simulink model "mc_att_control"  (R2024b)
settings: configuration reference "simulation" (kept outside this file)
undefined symbols (not defined in the file or in its folder): AIRMODE_ROLL_PITCH_YAW, deg, DiscIntNeverNeededParam, MC_ACRO_EXPO, MC_ACRO_EXPO_Y, MC_ACRO_P_MAX, MC_ACRO_R_MAX, MC_ACRO_SUPEXPO, MC_ACRO_SUPEXPOY, MC_ACRO_Y_MAX, MC_AIRMODE, MC_BAT_SCALE_EN, MC_MAN_TILT_TAU, MC_PITCH_P, MC_PITCHRATE_D, MC_PITCHRATE_FF, MC_PITCHRATE_I, MC_PITCHRATE_K, MC_PITCHRATE_MAX, MC_PITCHRATE_P, MC_PR_INT_LIM, MC_ROLL_P, MC_ROLLRATE_D, MC_ROLLRATE_FF, MC_ROLLRATE_I, MC_ROLLRATE_K, MC_ROLLRATE_MAX, MC_ROLLRATE_P, MC_RR_INT_LIM, MC_YAW_P, MC_YAW_WEIGHT, MC_YAWRATE_D, MC_YAWRATE_FF, MC_YAWRATE_I, MC_YAWRATE_K, MC_YAWRATE_MAX, MC_YAWRATE_P, MC_YR_INT_LIM, MPC_MAN_TILT_MAX, MPC_MAN_Y_MAX, MPC_MANTHR_MIN, MPC_THR_CURVE, MPC_THR_HOVER, MPC_THR_MAX, param_mpc_thr_hover, param_mpc_thr_max, rad, s, VEHICLE_TYPE_ROTARY_WING
libraries: simulink x22, aerolibutil x11, sharedtransform x4, aerolibconvert2 x3, vrlib x2, sharedutil x1
(part 1 of 2)
settings Model: DataDictionary=nextpilot_datadict.sldd  Creator=DELL  LastModifiedBy=93114
settings ConfigSetRef: SourceName=simulation

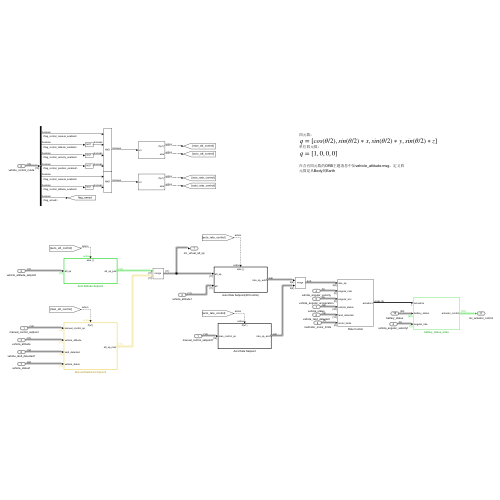
[thumbnail: Simulink's stored preview of the top-level diagram]
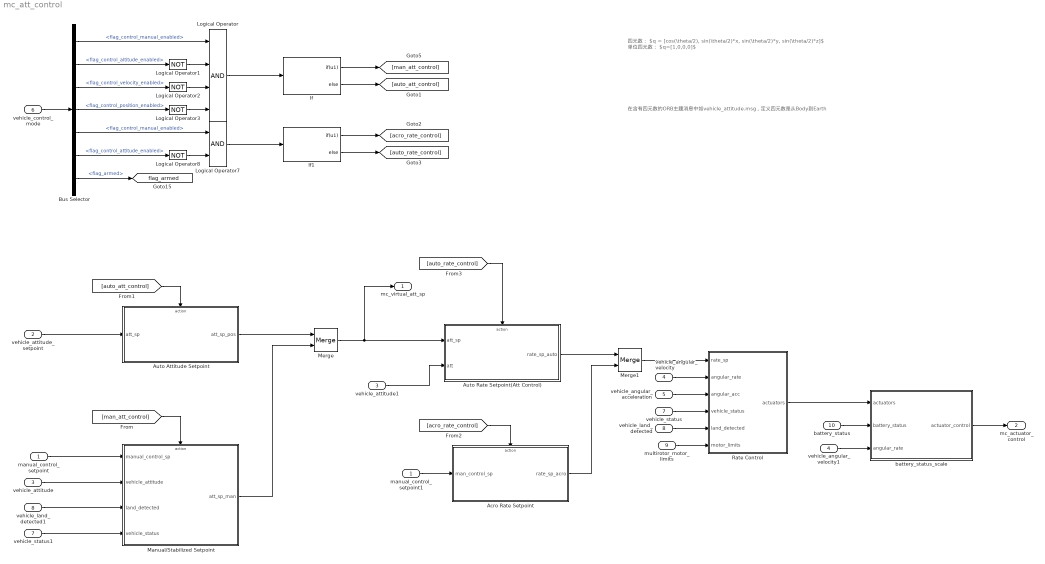
== system mc_att_control ==
  note: 在含有四元数的ORB主题消息中如vehicle_attitude.msg，定义四元数是从Body到Earth
  note: 四元数：
      | $q = [cos(\theta/2), sin(\theta/2)*x, sin(\theta/2)*y, sin(\theta/2)*z]$
      | 单位四元数：
      | $q=[1,0,0,0]$
  manual_control_setpoint : Inport  OutDataTypeStr=Bus: manual_control_setpoint_s
  vehicle_attitude_setpoint : Inport  Port=2  OutDataTypeStr=Bus: vehicle_attitude_setpoint_s
  vehicle_attitude : Inport  Port=3  OutDataTypeStr=Bus: vehicle_attitude_s
  vehicle_angular_velocity : Inport  Port=4  OutDataTypeStr=Bus: vehicle_angular_velocity_s
  vehicle_angular_acceleration : Inport  Port=5  OutDataTypeStr=Bus: vehicle_angular_acceleration_s
  vehicle_control_mode : Inport  Port=6  OutDataTypeStr=Bus: vehicle_control_mode_s
  vehicle_status : Inport  Port=7  OutDataTypeStr=Bus: vehicle_status_s
  vehicle_land_detected : Inport  Port=8  OutDataTypeStr=Bus: vehicle_land_detected_s
  multirotor_motor_limits : Inport  Port=9  OutDataTypeStr=Bus: multirotor_motor_limits_s
  battery_status : Inport  Port=10  OutDataTypeStr=Bus: battery_status_s
  Acro Rate Setpoint : Subsystem
  Auto Attitude Setpoint : Subsystem
  Auto Rate Setpoint(Att Control) : Subsystem
  Bus Selector : BusSelector  OutputSignals=flag_control_manual_enabled,flag_control_altitude_enabled,flag_control_velocity_enabled,flag_control_position_enabled,flag_control_manual_enabled,flag_control_attitude_enabled,flag_armed
  If : If  IfExpression=u1
  If1 : If  IfExpression=u1
  Logical Operator : Logic  Inputs=4  AllPortsSameDT=off  OutDataTypeStr=boolean
  Logical Operator{1..3,8} (4 alike) : Logic  Operator=NOT  Inputs=4  AllPortsSameDT=off  OutDataTypeStr=boolean
  Logical Operator7 : Logic  AllPortsSameDT=off  OutDataTypeStr=boolean
  Manual/Stabilized Setpoint : Subsystem
  Merge : Merge
  Merge1 : Merge
  Rate Control : Subsystem
  battery_status_scale : Subsystem
  manual_control_setpoint1 : InportShadow  OutDataTypeStr=Bus: manual_control_setpoint_s
  vehicle_angular_velocity1 : InportShadow  Port=4  OutDataTypeStr=Bus: vehicle_angular_velocity_s
  vehicle_attitude1 : InportShadow  Port=3  OutDataTypeStr=Bus: vehicle_attitude_s
  vehicle_land_detected1 : InportShadow  Port=8  OutDataTypeStr=Bus: vehicle_land_detected_s
  vehicle_status1 : InportShadow  Port=7  OutDataTypeStr=Bus: vehicle_status_s
  mc_virtual_att_sp : Outport  OutDataTypeStr=Bus: vehicle_attitude_setpoint_s  BusOutputAsStruct=on
  mc_actuator_control : Outport  Port=2  OutDataTypeStr=Bus: actuator_controls_s  BusOutputAsStruct=on
  tag scope: flag_armed=global
  wires:
  manual_control_setpoint/1 -> Manual/Stabilized Setpoint/1(manual_control_sp)
  Bus Selector/1 -> Logical Operator/1  "<flag_control_manual_enabled>"
  Bus Selector/2 -> Logical Operator1/1  "<flag_control_altitude_enabled>"
  Bus Selector/3 -> Logical Operator2/1  "<flag_control_velocity_enabled>"
  Bus Selector/4 -> Logical Operator3/1  "<flag_control_position_enabled>"
  Logical Operator1/1 -> Logical Operator/2
  Logical Operator2/1 -> Logical Operator/3
  Logical Operator3/1 -> Logical Operator/4
  vehicle_attitude/1 -> Manual/Stabilized Setpoint/2(vehicle_attitude)
  Logical Operator8/1 -> Logical Operator7/2
  Logical Operator7/1 -> If1/1
  Auto Rate Setpoint(Att Control)/1(rate_sp_auto) -> Merge1/1
  Manual/Stabilized Setpoint/1(att_sp_man) -> Merge/2
  vehicle_attitude1/1 -> Auto Rate Setpoint(Att Control)/2(att)
  vehicle_land_detected1/1 -> Manual/Stabilized Setpoint/3(land_detected)
  If/1 -> [man_att_control]
  If/2 -> [auto_att_control]
  [man_att_control] -> Manual/Stabilized Setpoint/Action
  [auto_att_control] -> Auto Attitude Setpoint/Action
  vehicle_control_mode/1 -> Bus Selector/1
  If1/1 -> [acro_rate_control]
  If1/2 -> [auto_rate_control]
  [acro_rate_control] -> Acro Rate Setpoint/Action
  Bus Selector/5 -> Logical Operator7/1  "<flag_control_manual_enabled>"
  Bus Selector/6 -> Logical Operator8/1  "<flag_control_attitude_enabled>"
  Bus Selector/7 -> [flag_armed]  "<flag_armed>"
  vehicle_status/1 -> Rate Control/4(vehicle_status)
  vehicle_status1/1 -> Manual/Stabilized Setpoint/4(vehicle_status)
  manual_control_setpoint1/1 -> Acro Rate Setpoint/1(man_control_sp)
  vehicle_angular_velocity/1 -> Rate Control/2(angular_rate)
  vehicle_angular_acceleration/1 -> Rate Control/3(angular_acc)
  Acro Rate Setpoint/1(rate_sp_acro) -> Merge1/2
  [auto_rate_control] -> Auto Rate Setpoint(Att Control)/Action
  Merge1/1 -> Rate Control/1(rate_sp)
  Merge/1 -> mc_virtual_att_sp/1, Auto Rate Setpoint(Att Control)/1(att_sp)
  battery_status_scale/1(actuator_control) -> mc_actuator_control/1
  Rate Control/1(actuators) -> battery_status_scale/1(actuators)
  battery_status/1 -> battery_status_scale/2(battery_status)
  vehicle_angular_velocity1/1 -> battery_status_scale/3(angular_rate)
  Auto Attitude Setpoint/1(att_sp_pos) -> Merge/1
  vehicle_attitude_setpoint/1 -> Auto Attitude Setpoint/1(att_sp)
  Logical Operator/1 -> If/1
  multirotor_motor_limits/1 -> Rate Control/6(motor_limits)
  vehicle_land_detected/1 -> Rate Control/5(land_detected)

== system mc_att_control/Acro Rate Setpoint ==
  Bus Element In : Inport  PortName=man_control_sp
  Bus Element In1 : Inport  PortName=man_control_sp  Element=z
  Action Port : ActionPort  ActionPortLabel=if(u1)
  Angular Velocity Conversion : aerolibconvert2/Angular Velocity Conversion  IU=deg/s  OU=rad/s
  Constant : Constant  Value=MC_ACRO_R_MAX
  Constant1 : Constant  Value=MC_ACRO_P_MAX
  Constant2 : Constant  Value=MC_ACRO_Y_MAX
  Demux : Demux  Outputs=3
  Gain : Gain
  Gain1 : Gain
  Gain2 : Gain
  Mux : Mux  Inputs=3
  Product : Product
  Saturation : Saturate  UpperLimit=1.0  LowerLimit=0.0
      settings: AttributesFormatString=[%<LowerLimit>,%<UpperLimit>]
  Unary Minus : UnaryMinus
  superexpo : Subsystem
  Bus Element Out : Outport  PortName=rate_sp_acro  Element=roll_rate_sp
  Bus Element Out1 : Outport  PortName=rate_sp_acro  Element=pitch_rate_sp
  Bus Element Out2 : Outport  PortName=rate_sp_acro  Element=yaw_rate_sp
  Bus Element Out3 : Outport  PortName=rate_sp_acro  Element=thrust_sp
  wires:
  Bus Element In1/1 -> Saturation/1
  Saturation/1 -> Unary Minus/1
  superexpo/1(man_rate_sp) -> Product/1
  Constant1/1 -> Mux/2
  Constant/1 -> Mux/1
  Constant2/1 -> Mux/3
  Mux/1 -> Angular Velocity Conversion/1
  Angular Velocity Conversion/1 -> Product/2  "parameter"
  Bus Element In/1 -> superexpo/1(man_stick)
  Demux/1 -> Gain2/1
  Demux/2 -> Gain1/1
  Demux/3 -> Gain/1
  Unary Minus/1 -> Bus Element Out3/1
  Product/1 -> Demux/1
  Gain/1 -> Bus Element Out2/1
  Gain1/1 -> Bus Element Out1/1
  Gain2/1 -> Bus Element Out/1

== system mc_att_control/Auto Attitude Setpoint ==
  att_sp : Inport
  Action Port : ActionPort  ActionPortLabel=else
  att_sp_pos : Outport
  wires:
  att_sp/1 -> att_sp_pos/1

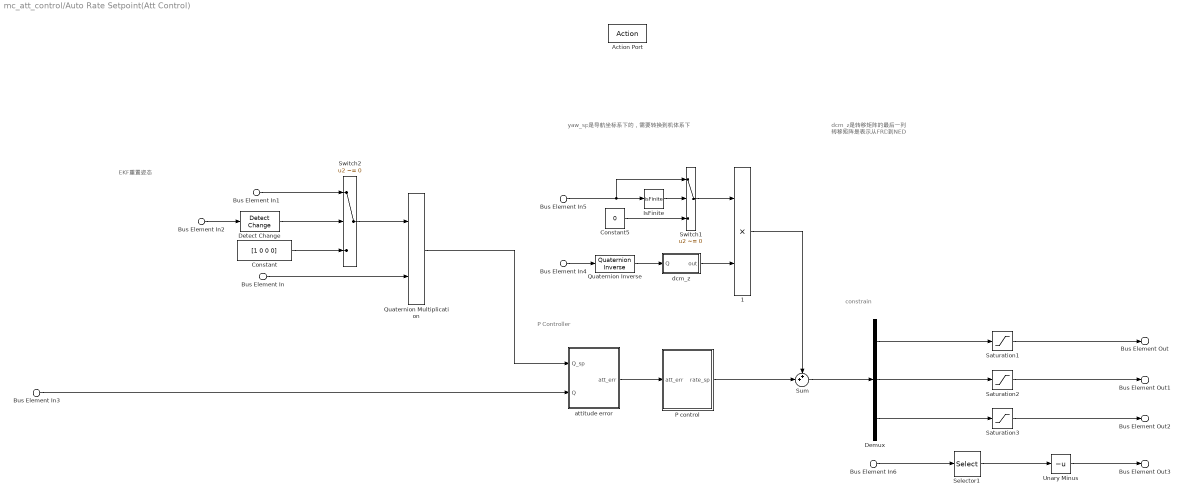
== system mc_att_control/Auto Rate Setpoint(Att Control) ==
  note: dcm_z是转移矩阵的最后一列
      | 转移矩阵是表示从FRD到NED
  note: constrain
  note: yaw_sp是导航坐标系下的，需要转换到机体系下
  note: EKF重置姿态
  note: P Controller
  Bus Element In : Inport  PortName=att_sp  Element=q_d
  Bus Element In5 : Inport  PortName=att_sp  Element=yaw_sp_move_rate
  Bus Element In6 : Inport  PortName=att_sp  Element=thrust_body
  Bus Element In1 : Inport  Port=2  PortName=att  Element=delta_q_reset
  Bus Element In2 : Inport  Port=2  PortName=att  Element=quat_reset_counter
  Bus Element In3 : Inport  Port=2  PortName=att  Element=q
  Bus Element In4 : Inport  Port=2  PortName=att  Element=q
  Action Port : ActionPort  ActionPortLabel=else
  1 : Product
  Constant : Constant  Value=[1 0 0 0]  OutDataTypeStr=single
  Constant5 : Constant  Value=0  OutDataTypeStr=single
  Demux : Demux  Outputs=3
  Detect Change : simulink/Logic and Bit Operations/Detect Change  vinit=0  OutDataTypeStr=boolean
  IsFinite : RelationalOperator  Operator=isFinite  OutDataTypeStr=boolean  RndMeth=Simplest  InputSameDT=off
  P control : Subsystem
  Quaternion Inverse : aerolibutil/Quaternion Inverse
  Quaternion Multiplication : aerolibutil/Quaternion Multiplication
  Saturation1 : Saturate  UpperLimit=deg2rad(MC_ROLLRATE_MAX)  LowerLimit=-deg2rad(MC_ROLLRATE_MAX)
      settings: AttributesFormatString=[%<LowerLimit>,%<UpperLimit>]
  Saturation2 : Saturate  UpperLimit=deg2rad(MC_PITCHRATE_MAX)  LowerLimit=-deg2rad(MC_PITCHRATE_MAX)
      settings: AttributesFormatString=[%<LowerLimit>,%<UpperLimit>]
  Saturation3 : Saturate  UpperLimit=deg2rad(MC_YAWRATE_MAX)  LowerLimit=-deg2rad(MC_YAWRATE_MAX)
      settings: AttributesFormatString=[%<LowerLimit>,%<UpperLimit>]
  Selector1 : Selector  InputPortWidth=3  IndexOptions=Index vector (dialog)  Indices=3  OutputSizes=1
  Sum : Sum  Inputs=++|
  Switch1 : Switch  Criteria=u2 ~= 0  SaturateOnIntegerOverflow=off  InputSameDT=off
  Switch2 : Switch  Criteria=u2 ~= 0  SaturateOnIntegerOverflow=off  InputSameDT=off
  Unary Minus : UnaryMinus
  attitude error : Subsystem
  dcm_z : Subsystem
  Bus Element Out : Outport  PortName=rate_sp_auto  Element=roll_rate_sp
  Bus Element Out1 : Outport  PortName=rate_sp_auto  Element=pitch_rate_sp
  Bus Element Out2 : Outport  PortName=rate_sp_auto  Element=yaw_rate_sp
  Bus Element Out3 : Outport  PortName=rate_sp_auto  Element=thrust_sp
  wires:
  P control/1(rate_sp) -> Sum/2
  Demux/1 -> Saturation1/1
  Demux/2 -> Saturation2/1
  Demux/3 -> Saturation3/1
  Saturation1/1 -> Bus Element Out/1
  Saturation2/1 -> Bus Element Out1/1
  Saturation3/1 -> Bus Element Out2/1
  Quaternion Multiplication/1 -> attitude error/1(Q_sp)
  Bus Element In3/1 -> attitude error/2(Q)
  Bus Element In4/1 -> Quaternion Inverse/1
  Quaternion Inverse/1 -> dcm_z/1(Q)
  dcm_z/1(out) -> 1/2
  Bus Element In5/1 -> Switch1/1, IsFinite/1
  1/1 -> Sum/1
  IsFinite/1 -> Switch1/2
  Constant5/1 -> Switch1/3
  Switch1/1 -> 1/1
  Detect Change/1 -> Switch2/2
  Switch2/1 -> Quaternion Multiplication/1
  Bus Element In/1 -> Quaternion Multiplication/2
  Constant/1 -> Switch2/3
  Bus Element In2/1 -> Detect Change/1
  Bus Element In1/1 -> Switch2/1
  Bus Element In6/1 -> Selector1/1
  Unary Minus/1 -> Bus Element Out3/1
  Sum/1 -> Demux/1
  Selector1/1 -> Unary Minus/1
  attitude error/1(att_err) -> P control/1(att_err)

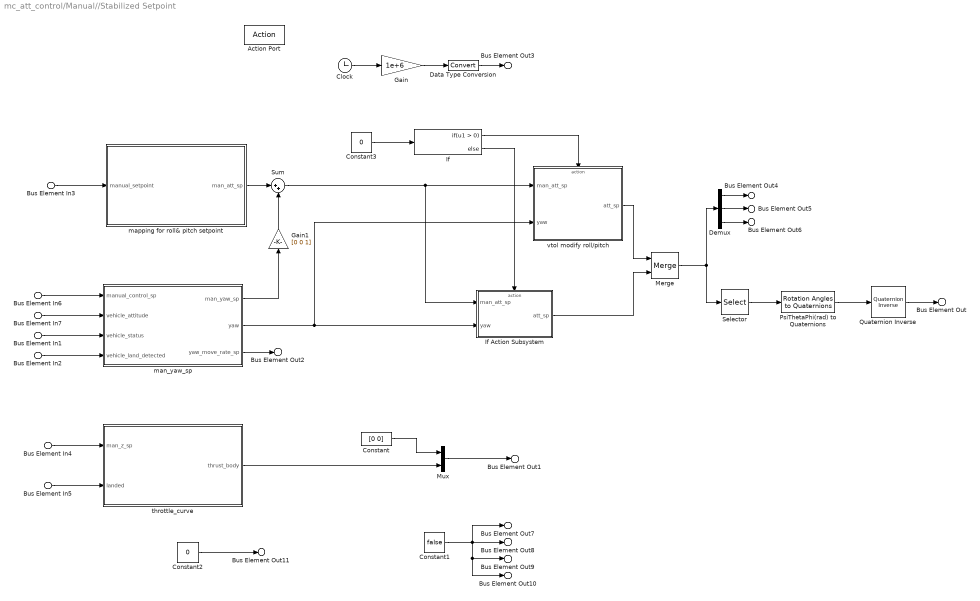
== system mc_att_control/Manual//Stabilized Setpoint ==
  Bus Element In6 : Inport  PortName=manual_control_sp
  Bus Element In3 : Inport  PortName=manual_control_sp
  Bus Element In4 : Inport  PortName=manual_control_sp  Element=z
  Bus Element In7 : Inport  Port=2  PortName=vehicle_attitude
  Bus Element In2 : Inport  Port=3  PortName=land_detected
  Bus Element In5 : Inport  Port=3  PortName=land_detected  Element=landed
  Bus Element In1 : Inport  Port=4  PortName=vehicle_status
  Action Port : ActionPort  InitializeStates=reset  ActionPortLabel=if(u1)
  Clock : Clock
  Constant : Constant  Value=[0 0]  OutDataTypeStr=single
  Constant1 : Constant  Value=false
  Constant2 : Constant  Value=0  OutDataTypeStr=uint8
  Constant3 : Constant  Value=0
  Data Type Conversion : DataTypeConversion  SaturateOnIntegerOverflow=off  RndMeth=Floor
  Demux : Demux  Outputs=3
  Gain : Gain  Gain=1e+6  OutDataTypeStr=uint64
      settings: AttributesFormatString=%<Gain>
  Gain1 : Gain  Gain=[0 0 1]
  If : If
  If Action Subsystem : Subsystem  TreatAsAtomicUnit=on
  Merge : Merge
  Mux : Mux  Inputs=2
  PsiThetaPhi(rad) to Quaternions : sharedtransform/Rotation Angles to Quaternions  rotationOrder=ZYX  aMode=aMode
  Quaternion Inverse : aerolibutil/Quaternion Inverse
  Selector : Selector  InputPortWidth=3  IndexOptions=Index vector (dialog)  Indices=[3 2 1]  OutputSizes=1
  Sum : Sum  Inputs=|++
  man_yaw_sp : Subsystem
  mapping for roll& pitch setpoint : Subsystem
  throttle_curve : Subsystem
  vtol modify roll/pitch : Subsystem
  Bus Element Out3 : Outport  PortName=att_sp_man  Element=timestamp
  Bus Element Out4 : Outport  PortName=att_sp_man  Element=roll_body
  Bus Element Out5 : Outport  PortName=att_sp_man  Element=pitch_body
  Bus Element Out6 : Outport  PortName=att_sp_man  Element=yaw_body
  Bus Element Out2 : Outport  PortName=att_sp_man  Element=yaw_sp_move_rate
  Bus Element Out : Outport  PortName=att_sp_man  Element=q_d
  Bus Element Out1 : Outport  PortName=att_sp_man  Element=thrust_body
  Bus Element Out7 : Outport  PortName=att_sp_man  Element=roll_reset_integral
  Bus Element Out8 : Outport  PortName=att_sp_man  Element=pitch_reset_integral
  Bus Element Out9 : Outport  PortName=att_sp_man  Element=yaw_reset_integral
  Bus Element Out10 : Outport  PortName=att_sp_man  Element=fw_control_yaw
  Bus Element Out11 : Outport  PortName=att_sp_man  Element=apply_flaps
  wires:
  Bus Element In4/1 -> throttle_curve/1(man_z_sp)
  Bus Element In5/1 -> throttle_curve/2(landed)
  throttle_curve/1(thrust_body) -> Mux/2
  Bus Element In7/1 -> man_yaw_sp/2(vehicle_attitude)
  Bus Element In1/1 -> man_yaw_sp/3(vehicle_status)
  Clock/1 -> Gain/1
  Gain/1 -> Data Type Conversion/1
  Constant/1 -> Mux/1
  Mux/1 -> Bus Element Out1/1
  Constant1/1 -> Bus Element Out10/1, Bus Element Out9/1, Bus Element Out7/1, Bus Element Out8/1
  Constant2/1 -> Bus Element Out11/1
  Data Type Conversion/1 -> Bus Element Out3/1
  Bus Element In2/1 -> man_yaw_sp/4(vehicle_land_detected)
  Bus Element In6/1 -> man_yaw_sp/1(manual_control_sp)
  Bus Element In3/1 -> mapping for roll& pitch setpoint/1(manual_setpoint)
  man_yaw_sp/3(yaw_move_rate_sp) -> Bus Element Out2/1
  If/1 -> vtol modify roll/pitch/Action
  If/2 -> If Action Subsystem/Action
  Constant3/1 -> If/1
  man_yaw_sp/1(man_yaw_sp) -> Gain1/1
  Gain1/1 -> Sum/2
  mapping for roll& pitch setpoint/1(man_att_sp) -> Sum/1
  man_yaw_sp/2(yaw) -> vtol modify roll/pitch/2(yaw), If Action Subsystem/2(yaw)
  Sum/1 -> If Action Subsystem/1(man_att_sp), vtol modify roll/pitch/1(man_att_sp)
  If Action Subsystem/1(att_sp) -> Merge/2
  PsiThetaPhi(rad) to Quaternions/1 -> Quaternion Inverse/1
  vtol modify roll/pitch/1(att_sp) -> Merge/1
  Merge/1 -> Selector/1, Demux/1
  Selector/1 -> PsiThetaPhi(rad) to Quaternions/1
  Quaternion Inverse/1 -> Bus Element Out/1
  Demux/3 -> Bus Element Out6/1
  Demux/2 -> Bus Element Out5/1
  Demux/1 -> Bus Element Out4/1

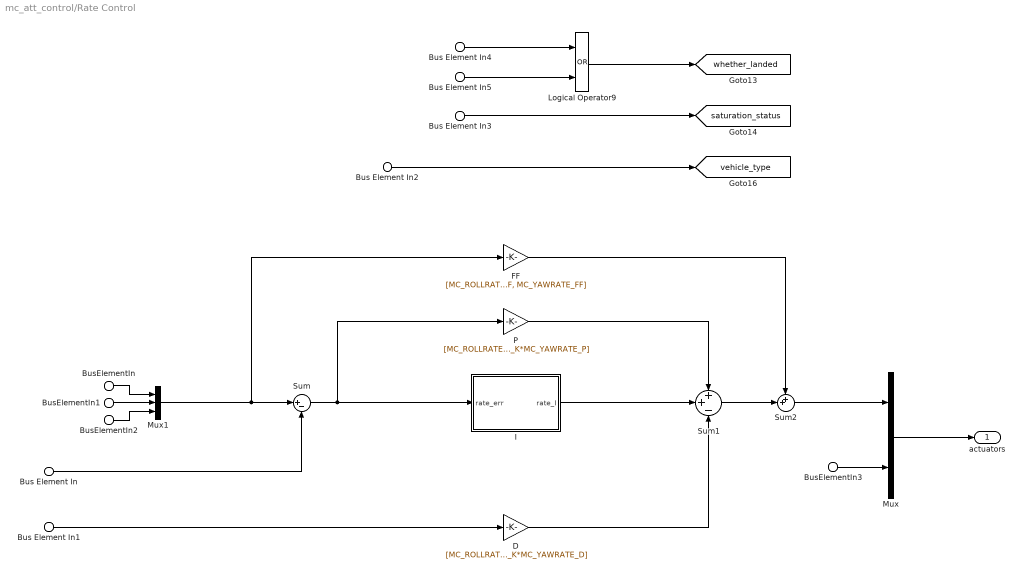
== system mc_att_control/Rate Control ==
  BusElementIn : Inport  PortName=rate_sp  Element=roll_rate_sp
  BusElementIn1 : Inport  PortName=rate_sp  Element=pitch_rate_sp
  BusElementIn2 : Inport  PortName=rate_sp  Element=yaw_rate_sp
  BusElementIn3 : Inport  PortName=rate_sp  Element=thrust_sp
  Bus Element In : Inport  Port=2  PortName=angular_rate  Element=xyz
  Bus Element In1 : Inport  Port=3  PortName=angular_acc  Element=xyz
  Bus Element In2 : Inport  Port=4  PortName=vehicle_status  Element=vehicle_type
  Bus Element In4 : Inport  Port=5  PortName=land_detected  Element=landed
  Bus Element In5 : Inport  Port=5  PortName=land_detected  Element=maybe_landed
  Bus Element In3 : Inport  Port=6  PortName=motor_limits  Element=saturation_status
  D : Gain  Gain=[MC_ROLLRATE_K*MC_ROLLRATE_D MC_PITCHRATE_K*MC_PITCHRATE_D MC_YAWRATE_K*MC_YAWRATE_D]
      settings: AttributesFormatString=%<Gain>
  FF : Gain  Gain=[MC_ROLLRATE_FF, MC_PITCHRATE_FF, MC_YAWRATE_FF]
      settings: AttributesFormatString=%<Gain>
  I : Subsystem
  Logical Operator9 : Logic  Operator=OR  AllPortsSameDT=off  OutDataTypeStr=boolean
  Mux : Mux  Inputs=2
  Mux1 : Mux  Inputs=3
  P : Gain  Gain=[MC_ROLLRATE_K*MC_ROLLRATE_P, MC_PITCHRATE_K*MC_PITCHRATE_P, MC_YAWRATE_K*MC_YAWRATE_P]
      settings: AttributesFormatString=%<Gain>
  Sum : Sum  Inputs=|+-
  Sum1 : Sum  Inputs=++-
  Sum2 : Sum  Inputs=++|
  actuators : Outport
  tag scope: saturation_status=global, vehicle_type=global, whether_landed=global
  wires:
  Bus Element In/1 -> Sum/2
  FF/1 -> Sum2/1
  P/1 -> Sum1/1
  Sum/1 -> I/1(rate_err), P/1
  I/1(rate_I) -> Sum1/2
  D/1 -> Sum1/3
  Sum1/1 -> Sum2/2
  Bus Element In1/1 -> D/1
  Mux1/1 -> FF/1, Sum/1
  Mux/1 -> actuators/1
  Sum2/1 -> Mux/1
  Logical Operator9/1 -> [whether_landed]
  Bus Element In4/1 -> Logical Operator9/1
  Bus Element In5/1 -> Logical Operator9/2
  Bus Element In2/1 -> [vehicle_type]
  Bus Element In3/1 -> [saturation_status]
  BusElementIn1/1 -> Mux1/2
  BusElementIn/1 -> Mux1/1
  BusElementIn2/1 -> Mux1/3
  BusElementIn3/1 -> Mux/2

== system mc_att_control/battery_status_scale ==
  actuators : Inport
  Bus Element In : Inport  Port=2  PortName=battery_status  Element=connected
  Bus Element In1 : Inport  Port=2  PortName=battery_status  Element=scale
  Bus Element In2 : Inport  Port=2  PortName=battery_status  Element=scale
  In Bus Element : Inport  Port=3  PortName=angular_rate  Element=timestamp_sample
  Clock : Clock
  Compare To Zero : simulink/Logic and Bit Operations/Compare To Zero  relop=>  OutDataTypeStr=boolean
  Constant : Constant  Value=MC_BAT_SCALE_EN  OutDataTypeStr=boolean
  Constant1 : Constant  OutDataTypeStr=single
  Constant2 : Constant  Value=[0 0 0 0]  OutDataTypeStr=single
  Gain : Gain  Gain=1e+6  OutDataTypeStr=uint64
      settings: AttributesFormatString=%<Gain>
  Logical Operator : Logic  Inputs=3  AllPortsSameDT=off  OutDataTypeStr=boolean
  Mux : Mux  Inputs=2
  Product : Product
  Switch : Switch  Criteria=u2 ~= 0  SaturateOnIntegerOverflow=off  InputSameDT=off
  Bus Element Out1 : Outport  PortName=actuator_control  Element=timestamp
  Bus Element Out2 : Outport  PortName=actuator_control  Element=timestamp_sample
  Bus Element Out4 : Outport  PortName=actuator_control  Element=control
  wires:
  Constant/1 -> Logical Operator/1
  Bus Element In/1 -> Logical Operator/2
  Compare To Zero/1 -> Logical Operator/3
  Bus Element In1/1 -> Compare To Zero/1
  Logical Operator/1 -> Switch/2
  Bus Element In2/1 -> Switch/1
  Constant1/1 -> Switch/3
  Switch/1 -> Product/2
  actuators/1 -> Product/1
  Gain/1 -> Bus Element Out1/1
  Product/1 -> Mux/1
  Constant2/1 -> Mux/2
  Mux/1 -> Bus Element Out4/1
  Clock/1 -> Gain/1
  In Bus Element/1 -> Bus Element Out2/1

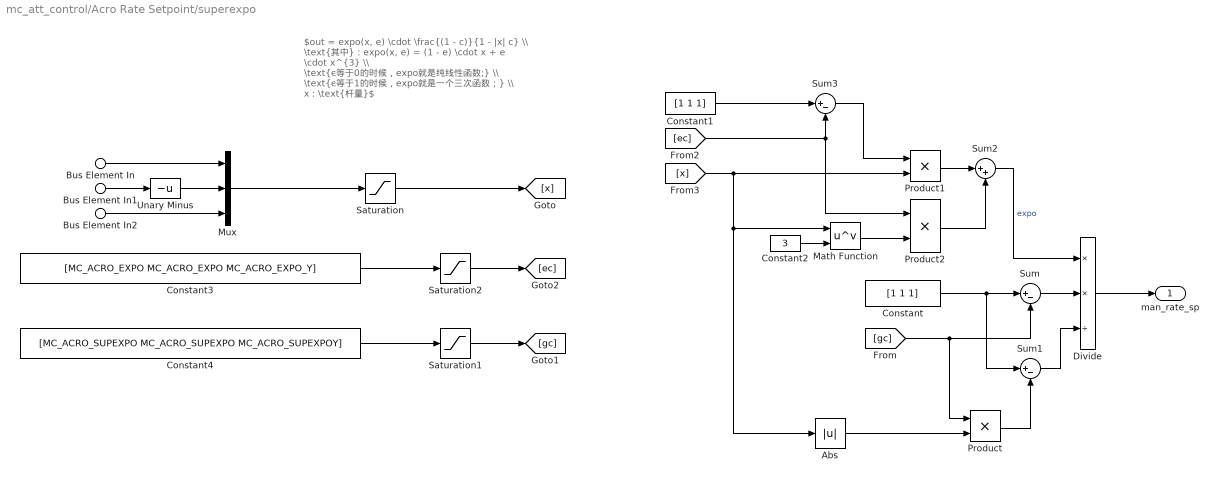
== system mc_att_control/Acro Rate Setpoint/superexpo ==
  note: $out = expo(x, e) \cdot \frac{(1 - c)}{1 - |x| c} \\ \text{其中}：expo(x, e) = (1 - e) \cdot x + e \cdot x^{3} \\ \text{e等于0的时候，expo就是纯线性函数;} \\ \text{e等于1的时候，expo就是一个三次函数；} \\ x：\text{杆量}$
  Bus Element In : Inport  PortName=man_stick  Element=y
  Bus Element In1 : Inport  PortName=man_stick  Element=x
  Bus Element In2 : Inport  PortName=man_stick  Element=r
  Abs : Abs  SaturateOnIntegerOverflow=off
  Constant : Constant  Value=[1 1 1]  OutDataTypeStr=single
  Constant1 : Constant  Value=[1 1 1]  OutDataTypeStr=single
  Constant2 : Constant  Value=3  OutDataTypeStr=single
  Constant3 : Constant  Value=[MC_ACRO_EXPO MC_ACRO_EXPO MC_ACRO_EXPO_Y]
  Constant4 : Constant  Value=[MC_ACRO_SUPEXPO MC_ACRO_SUPEXPO MC_ACRO_SUPEXPOY]
  Divide : Product  Inputs=**/
  Math Function : Math  Operator=pow
  Mux : Mux  Inputs=3
  Product : Product
  Product1 : Product
  Product2 : Product
  Saturation : Saturate  UpperLimit=1.0  LowerLimit=-1.0
      settings: AttributesFormatString=[%<LowerLimit>,%<UpperLimit>]
  Saturation1 : Saturate  UpperLimit=single(0.99)  LowerLimit=0.0
      settings: AttributesFormatString=[%<LowerLimit>,%<UpperLimit>]
  Saturation2 : Saturate  UpperLimit=1.0  LowerLimit=0.0
      settings: AttributesFormatString=[%<LowerLimit>,%<UpperLimit>]
  Sum : Sum  Inputs=|+-
  Sum1 : Sum  Inputs=|+-
  Sum2 : Sum  Inputs=|++
  Sum3 : Sum  Inputs=|+-
  Unary Minus : UnaryMinus
  man_rate_sp : Outport
  wires:
  Saturation/1 -> [x]
  Constant4/1 -> Saturation1/1
  Saturation1/1 -> [gc]
  Divide/1 -> man_rate_sp/1
  Sum2/1 -> Divide/1  "expo"
  Sum/1 -> Divide/2
  Constant/1 -> Sum1/1, Sum/1
  [gc] -> Product/1, Sum/2
  Sum1/1 -> Divide/3
  [x] -> Abs/1, Math Function/1, Product1/2
  Abs/1 -> Product/2
  Product/1 -> Sum1/2
  Constant3/1 -> Saturation2/1
  Saturation2/1 -> [ec]
  Product1/1 -> Sum2/1
  Product2/1 -> Sum2/2
  Sum3/1 -> Product1/1
  Constant1/1 -> Sum3/1
  [ec] -> Product2/1, Sum3/2
  Math Function/1 -> Product2/2
  Constant2/1 -> Math Function/2
  Bus Element In/1 -> Mux/1
  Unary Minus/1 -> Mux/2
  Bus Element In1/1 -> Unary Minus/1
  Bus Element In2/1 -> Mux/3
  Mux/1 -> Saturation/1

== system mc_att_control/Auto Rate Setpoint(Att Control)/P control ==
  note: 姿态误差乘以比例系数，就是角速度环的期望值
  att_err : Inport
  Constant : Constant  Value=MC_ROLL_P
  Constant1 : Constant  Value=MC_PITCH_P
  Constant2 : Constant  Value=MC_YAW_P
  Constant3 : Constant  Value=MC_YAW_WEIGHT  OutDataTypeStr=single
  Constant4 : Constant  OutDataTypeStr=single
  Divide : Product  Inputs=*/
  Mux : Mux  Inputs=3
  Product : Product
  Saturation : Saturate  UpperLimit=1.0  LowerLimit=0.0
      settings: AttributesFormatString=[%<LowerLimit>,%<UpperLimit>]
  Switch : Switch  Criteria=u2 > Threshold  Threshold=single(1e-4)  SaturateOnIntegerOverflow=off  InputSameDT=off
      settings: AttributesFormatString=|
      | %<Criteria>
      | %<Threshold>
  rate_sp : Outport
  wires:
  Saturation/1 -> Switch/2, Switch/1
  Constant1/1 -> Mux/2
  Constant2/1 -> Divide/1
  Switch/1 -> Divide/2
  Constant/1 -> Mux/1
  Constant4/1 -> Switch/3
  Divide/1 -> Mux/3
  Constant3/1 -> Saturation/1
  Mux/1 -> Product/2
  att_err/1 -> Product/1
  Product/1 -> rate_sp/1

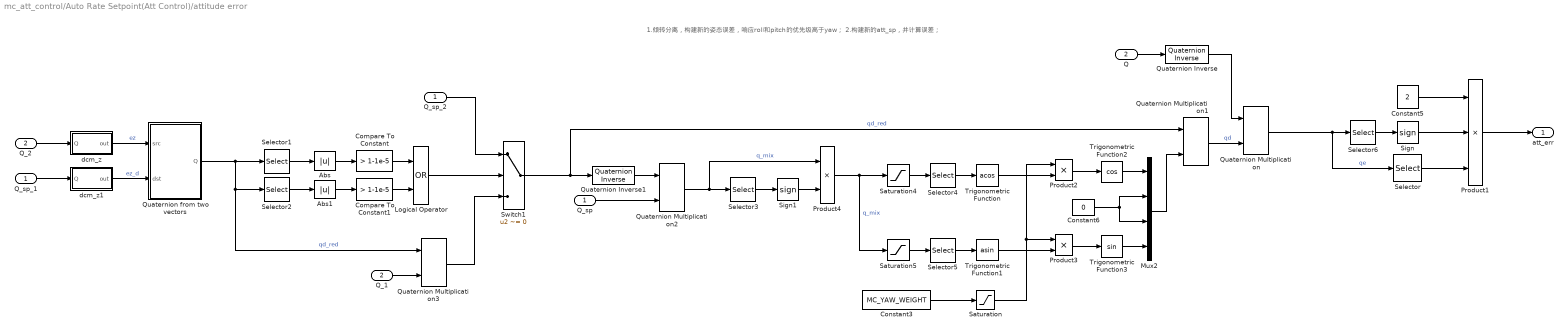
== system mc_att_control/Auto Rate Setpoint(Att Control)/attitude error ==
  note: 1.倾转分离，构建新的姿态误差，响应roll和pitch的优先级高于yaw；
      | 2.构建新的att_sp，并计算误差；
  Q_sp : Inport
  Q : Inport  Port=2
  Abs : Abs  SaturateOnIntegerOverflow=off
  Abs1 : Abs  SaturateOnIntegerOverflow=off
  Compare To Constant : simulink/Logic and Bit Operations/Compare To Constant  relop=>  const=1-1e-5  OutDataTypeStr=boolean
  Compare To Constant1 : simulink/Logic and Bit Operations/Compare To Constant  relop=>  const=1-1e-5  OutDataTypeStr=boolean
  Constant3 : Constant  Value=MC_YAW_WEIGHT  OutDataTypeStr=single
  Constant5 : Constant  Value=2  OutDataTypeStr=single
  Constant6 : Constant  Value=0  OutDataTypeStr=single
  Logical Operator : Logic  Operator=OR  AllPortsSameDT=off  OutDataTypeStr=boolean
  Mux2 : Mux
  Product1 : Product  Inputs=3
  Product2 : Product
  Product3 : Product
  Product4 : Product
  Q_1 : InportShadow  Port=2
  Q_2 : InportShadow  Port=2
  Q_sp_1 : InportShadow
  Q_sp_2 : InportShadow
  Quaternion Inverse : aerolibutil/Quaternion Inverse
  Quaternion Inverse1 : aerolibutil/Quaternion Inverse
  Quaternion Multiplication{,1..3} (4 alike) : aerolibutil/Quaternion Multiplication
  Quaternion from two vectors : Subsystem
  Saturation : Saturate  UpperLimit=1.0  LowerLimit=0.0
      settings: AttributesFormatString=[%<LowerLimit>,%<UpperLimit>]
  Saturation4 : Saturate  UpperLimit=1.0  LowerLimit=-1.0
  Saturation5 : Saturate  UpperLimit=1.0  LowerLimit=-1.0
  Selector : Selector  InputPortWidth=4  IndexOptions=Index vector (dialog)  Indices=[2 3 4]  OutputSizes=1
  Selector1 : Selector  InputPortWidth=4  IndexOptions=Index vector (dialog)  Indices=2  OutputSizes=1
  Selector2 : Selector  InputPortWidth=4  IndexOptions=Index vector (dialog)  Indices=3  OutputSizes=1
  Selector3 : Selector  InputPortWidth=4  IndexOptions=Index vector (dialog)  Indices=1  OutputSizes=1
  Selector4 : Selector  InputPortWidth=4  IndexOptions=Index vector (dialog)  Indices=1  OutputSizes=1
  Selector5 : Selector  InputPortWidth=4  IndexOptions=Index vector (dialog)  Indices=4  OutputSizes=1
  Selector6 : Selector  InputPortWidth=4  IndexOptions=Index vector (dialog)  Indices=1  OutputSizes=1
  Sign : Signum
  Sign1 : Signum
  Switch1 : Switch  Criteria=u2 ~= 0  SaturateOnIntegerOverflow=off  InputSameDT=off
  Trigonometric Function : Trigonometry  Operator=acos
  Trigonometric Function1 : Trigonometry  Operator=asin
  Trigonometric Function2 : Trigonometry  Operator=cos
  Trigonometric Function3 : Trigonometry
  dcm_z : Subsystem
  dcm_z1 : Subsystem
  att_err : Outport
  wires:
  Quaternion Multiplication2/1 -> Selector3/1, Product4/1  "q_mix"
  Product4/1 -> Saturation4/1, Saturation5/1  "q_mix"
  Selector4/1 -> Trigonometric Function/1
  Selector3/1 -> Sign1/1
  dcm_z1/1(out) -> Quaternion from two vectors/2(dst)  "ez_d"
  Quaternion Multiplication/1 -> Selector6/1, Selector/1  "qe"
  Quaternion Multiplication3/1 -> Switch1/3
  Switch1/1 -> Quaternion Multiplication1/1, Quaternion Inverse1/1  "qd_red"
  Q_sp_1/1 -> dcm_z1/1(Q)
  Trigonometric Function3/1 -> Mux2/4
  Q_sp_2/1 -> Switch1/1
  Saturation/1 -> Product2/1, Product3/1
  Abs/1 -> Compare To Constant/1
  Quaternion Multiplication1/1 -> Quaternion Multiplication/2  "qd"
  Trigonometric Function2/1 -> Mux2/1
  Constant5/1 -> Product1/1
  Q_1/1 -> Quaternion Multiplication3/2
  Q_sp/1 -> Quaternion Multiplication2/2
  Mux2/1 -> Quaternion Multiplication1/2
  Trigonometric Function1/1 -> Product3/2
  Selector2/1 -> Abs1/1
  Q_2/1 -> dcm_z/1(Q)
  Saturation4/1 -> Selector4/1
  Quaternion from two vectors/1(Q) -> Selector1/1, Selector2/1, Quaternion Multiplication3/1  "qd_red"
  Q/1 -> Quaternion Inverse/1
  Constant6/1 -> Mux2/2, Mux2/3
  Product2/1 -> Trigonometric Function2/1
  Selector6/1 -> Sign/1
  Selector1/1 -> Abs/1
  Selector5/1 -> Trigonometric Function1/1
  Quaternion Inverse1/1 -> Quaternion Multiplication2/1
  Trigonometric Function/1 -> Product2/2
  Sign1/1 -> Product4/2
  Saturation5/1 -> Selector5/1
  Logical Operator/1 -> Switch1/2
  Selector/1 -> Product1/3
  Quaternion Inverse/1 -> Quaternion Multiplication/1
  Abs1/1 -> Compare To Constant1/1
  dcm_z/1(out) -> Quaternion from two vectors/1(src)  "ez"
  Sign/1 -> Product1/2
  Compare To Constant/1 -> Logical Operator/1
  Compare To Constant1/1 -> Logical Operator/2
  Product3/1 -> Trigonometric Function3/1
  Constant3/1 -> Saturation/1
  Product1/1 -> att_err/1

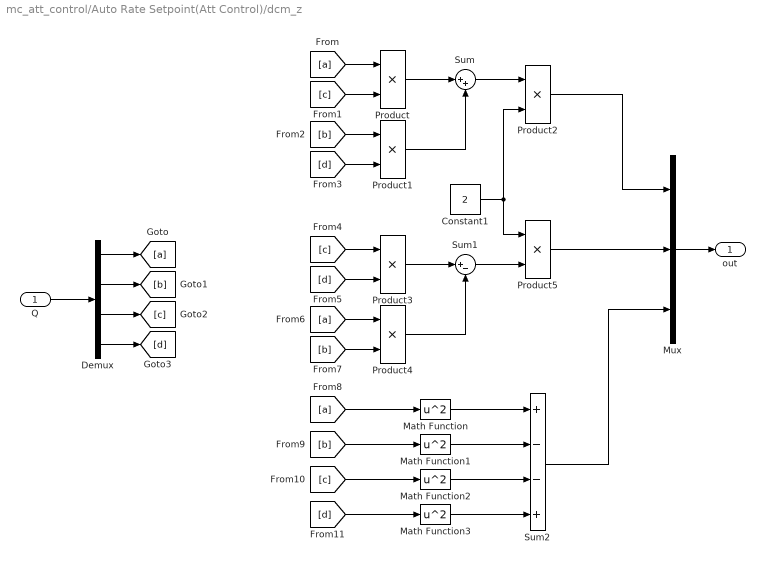
== system mc_att_control/Auto Rate Setpoint(Att Control)/dcm_z ==
  Q : Inport
  Constant1 : Constant  Value=2  OutDataTypeStr=single
  Demux : Demux
  Math Function{,1..3} (4 alike) : Math  Operator=square
  Mux : Mux  Inputs=3
  Product{,1..5} (6 alike) : Product
  Sum : Sum  Inputs=|++
  Sum1 : Sum  Inputs=|+-
  Sum2 : Sum  Inputs=+--+
  out : Outport
  wires:
  Q/1 -> Demux/1
  Demux/1 -> [a]
  Demux/2 -> [b]
  Demux/3 -> [c]
  Demux/4 -> [d]
  [a] -> Product/1
  [c] -> Product/2
  Product/1 -> Sum/1
  [b] -> Product1/1
  [d] -> Product1/2
  Product1/1 -> Sum/2
  Sum/1 -> Product2/1
  Product2/1 -> Mux/1
  Mux/1 -> out/1
  [c] -> Product3/1
  [d] -> Product3/2
  Product3/1 -> Sum1/1
  [a] -> Product4/1
  [b] -> Product4/2
  Product4/1 -> Sum1/2
  Sum1/1 -> Product5/2
  Constant1/1 -> Product5/1, Product2/2
  Product5/1 -> Mux/2
  Sum2/1 -> Mux/3
  [a] -> Math Function/1
  [b] -> Math Function1/1
  [c] -> Math Function2/1
  [d] -> Math Function3/1
  Math Function/1 -> Sum2/1
  Math Function1/1 -> Sum2/2
  Math Function2/1 -> Sum2/3
  Math Function3/1 -> Sum2/4

== system mc_att_control/Manual//Stabilized Setpoint/If Action Subsystem ==
  man_att_sp : Inport
  yaw : Inport  Port=2
  Action Port : ActionPort  ActionPortLabel=else
  Terminator : Terminator
  att_sp : Outport
  wires:
  man_att_sp/1 -> att_sp/1
  yaw/1 -> Terminator/1

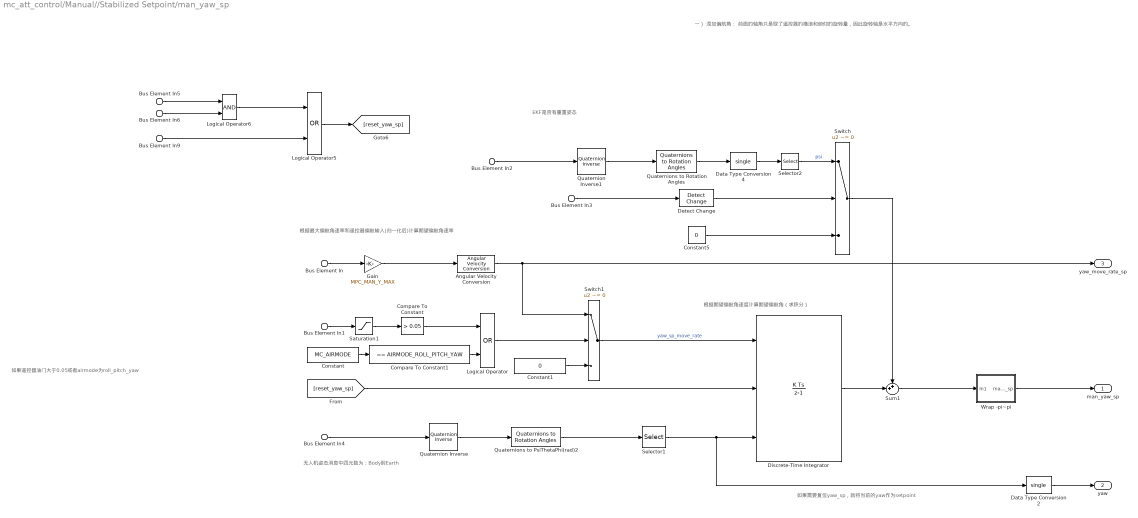
== system mc_att_control/Manual//Stabilized Setpoint/man_yaw_sp ==
  note: 无人机姿态消息中四元数为：Body到Earth
  note: 根据期望偏航角速度计算期望偏航角（求积分）
  note: 根据最大偏航角速率和遥控器偏航输入(归一化后)计算期望偏航角速率
  note: 如果遥控器油门大于0.05或者airmode为roll_pitch_yaw
  note: EKF是否有重置姿态
  note: 如果需要复位yaw_sp，就将当前的yaw作为setpoint
  note: 一） 添加偏航角：
      | 前面的轴角只是取了遥控器的横滚和俯仰的旋转量，因此旋转轴是水平方向的。
  Bus Element In : Inport  PortName=manual_control_sp  Element=r
  Bus Element In1 : Inport  PortName=manual_control_sp  Element=z
  Bus Element In2 : Inport  Port=2  PortName=vehicle_attitude  Element=delta_q_reset
  Bus Element In3 : Inport  Port=2  PortName=vehicle_attitude  Element=quat_reset_counter
  Bus Element In4 : Inport  Port=2  PortName=vehicle_attitude  Element=q
  Bus Element In5 : Inport  Port=3  PortName=vehicle_status  Element=is_vtol
  Bus Element In6 : Inport  Port=3  PortName=vehicle_status  Element=in_transition_mode
  Bus Element In9 : Inport  Port=4  PortName=vehicle_land_detected  Element=landed
  Angular Velocity Conversion : aerolibconvert2/Angular Velocity Conversion  IU=deg/s  OU=rad/s
  Compare To Constant : simulink/Logic and Bit Operations/Compare To Constant  relop=>  const=0.05  OutDataTypeStr=boolean
  Compare To Constant1 : simulink/Logic and Bit Operations/Compare To Constant  relop===  const=AIRMODE_ROLL_PITCH_YAW  OutDataTypeStr=boolean
  Constant : Constant  Value=MC_AIRMODE
  Constant1 : Constant  Value=0  OutDataTypeStr=single
  Constant5 : Constant  Value=0  OutDataTypeStr=single
  Data Type Conversion2 : DataTypeConversion  OutDataTypeStr=single  SaturateOnIntegerOverflow=off  RndMeth=Floor
  Data Type Conversion4 : DataTypeConversion  OutDataTypeStr=single  SaturateOnIntegerOverflow=off  RndMeth=Floor
  Detect Change : simulink/Logic and Bit Operations/Detect Change  vinit=0  OutDataTypeStr=boolean
  Discrete-Time Integrator : DiscreteIntegrator  ExternalReset=level  InitialConditionSource=external  SampleTime=-1  LimitOutput=on  UpperSaturationLimit=pi  LowerSaturationLimit=-pi  ICPrevOutput=DiscIntNeverNeededParam  ICPrevScaledInput=DiscIntNeverNeededParam
  Gain : Gain  Gain=MPC_MAN_Y_MAX
      settings: AttributesFormatString=%<Gain>
  Logical Operator : Logic  Operator=OR  AllPortsSameDT=off  OutDataTypeStr=boolean
  Logical Operator5 : Logic  Operator=OR  AllPortsSameDT=off  OutDataTypeStr=boolean
  Logical Operator6 : Logic  AllPortsSameDT=off  OutDataTypeStr=boolean
  Quaternion Inverse : aerolibutil/Quaternion Inverse
  Quaternion Inverse1 : aerolibutil/Quaternion Inverse
  Quaternions to PsiThetaPhi(rad)2 : sharedtransform/Quaternions to Rotation Angles  rotationOrder=ZYX  aMode=aMode
  Quaternions to Rotation Angles : sharedtransform/Quaternions to Rotation Angles  rotationOrder=ZYX  aMode=aMode
  Saturation1 : Saturate  UpperLimit=1  LowerLimit=0
      settings: AttributesFormatString=[%<LowerLimit>,%<UpperLimit>]
  Selector1 : Selector  InputPortWidth=3  IndexOptions=Index vector (dialog)  Indices=1  OutputSizes=1
  Selector2 : Selector  InputPortWidth=3  IndexOptions=Index vector (dialog)  Indices=1  OutputSizes=1
  Sum1 : Sum  Inputs=++|
  Switch : Switch  Criteria=u2 ~= 0  SaturateOnIntegerOverflow=off  InputSameDT=off
  Switch1 : Switch  Criteria=u2 ~= 0  SaturateOnIntegerOverflow=off  InputSameDT=off
  Wrap -pi~pi : Subsystem
  man_yaw_sp : Outport
  yaw : Outport  Port=2
  yaw_move_rate_sp : Outport  Port=3
  wires:
  Quaternions to PsiThetaPhi(rad)2/1 -> Selector1/1
  Quaternions to Rotation Angles/1 -> Data Type Conversion4/1
  Constant5/1 -> Switch/3
  Detect Change/1 -> Switch/2
  Gain/1 -> Angular Velocity Conversion/1
  Switch/1 -> Sum1/1
  Sum1/1 -> Wrap -pi~pi/1(In1)
  Selector1/1 -> Data Type Conversion2/1, Discrete-Time Integrator/3
  Angular Velocity Conversion/1 -> yaw_move_rate_sp/1, Switch1/1
  Discrete-Time Integrator/1 -> Sum1/2
  Selector2/1 -> Switch/1  "psi"
  [reset_yaw_sp] -> Discrete-Time Integrator/2
  Bus Element In/1 -> Gain/1
  Bus Element In3/1 -> Detect Change/1
  Switch1/1 -> Discrete-Time Integrator/1  "yaw_sp_move_rate"
  Bus Element In1/1 -> Saturation1/1
  Saturation1/1 -> Compare To Constant/1
  Compare To Constant/1 -> Logical Operator/1
  Constant/1 -> Compare To Constant1/1
  Logical Operator/1 -> Switch1/2
  Compare To Constant1/1 -> Logical Operator/2
  Logical Operator6/1 -> Logical Operator5/1
  Bus Element In6/1 -> Logical Operator6/2
  Logical Operator5/1 -> [reset_yaw_sp]
  Bus Element In9/1 -> Logical Operator5/2
  Bus Element In5/1 -> Logical Operator6/1
  Bus Element In4/1 -> Quaternion Inverse/1
  Bus Element In2/1 -> Quaternion Inverse1/1
  Data Type Conversion4/1 -> Selector2/1
  Quaternion Inverse/1 -> Quaternions to PsiThetaPhi(rad)2/1
  Quaternion Inverse1/1 -> Quaternions to Rotation Angles/1
  Constant1/1 -> Switch1/3
  Wrap -pi~pi/1(man_yaw_sp) -> man_yaw_sp/1
  Data Type Conversion2/1 -> yaw/1

== system mc_att_control/Manual//Stabilized Setpoint/mapping for roll& pitch setpoint ==
  note: 说明：本模块对应PX4的 MulticopterAttitudeControl::generate_attitude_setpoint()函数的前半部分
  note: 输入四元数为Earth转Body
  note: 二）计算横滚角、俯仰角期望
      | 1. roll和pitch通过遥控器的输入，用轴角法进行处理，进而生成setpoint；
      | 2. yaw通过遥控器的输入转换成yaw_sp，中间需要判断EFK端是否有重置yaw，需要加上delta_yaw；
  Bus Element In : Inport  PortName=manual_setpoint  Element=y
  Bus Element In1 : Inport  PortName=manual_setpoint  Element=x
  Angle Conversion : aerolibconvert2/Angle Conversion  IU=deg  OU=rad
  AxisAngle to Quat : Subsystem
  Gain : Gain  Gain=MPC_MAN_TILT_MAX
      settings: AttributesFormatString=%<Gain>
  Mux2 : Mux  Inputs=2
  Quaternions to PsiThetaPhi(rad) : sharedtransform/Quaternions to Rotation Angles  rotationOrder=ZYX  aMode=aMode
  Selector : Selector  InputPortWidth=3  IndexOptions=Index vector (dialog)  Indices=[3 2 1]  OutputSizes=1
  Unary Minus : UnaryMinus
  man_input_filter : Subsystem
  vector limitation : Subsystem
  man_att_sp : Outport
  wires:
  Gain/1 -> Angle Conversion/1
  Unary Minus/1 -> Mux2/2
  Mux2/1 -> Gain/1
  Angle Conversion/1 -> man_input_filter/1(man_sp)
  man_input_filter/1(output) -> vector limitation/1(v)
  Quaternions to PsiThetaPhi(rad)/1 -> Selector/1
  vector limitation/1(v_limited) -> AxisAngle to Quat/1(AxisAngle1)
  AxisAngle to Quat/1(Quat) -> Quaternions to PsiThetaPhi(rad)/1
  Bus Element In/1 -> Mux2/1
  Bus Element In1/1 -> Unary Minus/1
  Selector/1 -> man_att_sp/1

== system mc_att_control/Manual//Stabilized Setpoint/throttle_curve ==
  man_z_sp : Inport
  landed : Inport  Port=2
  1-D Lookup Table1 : Lookup_n-D  NumberOfTableDimensions=1  BreakpointsForDimension1=[0 0.5 1]  TableSource=Input port  Table=[param_mpc_thr_hover param_mpc_thr_max]  ExtrapMethod=Clip  UseLastTableValue=on  InternalRulePriority=Speed  RndMeth=Simplest
      settings: InputPortMap=u0,p221
  Compare To Constant : simulink/Logic and Bit Operations/Compare To Constant  relop===  const=1  OutDataTypeStr=boolean
  Constant1 : Constant  Value=MPC_MANTHR_MIN
  Constant2 : Constant  Value=MPC_THR_CURVE  OutDataTypeStr=int32
  Constant3 : Constant  Value=MPC_THR_MAX
  Constant4 : Constant  Value=MPC_THR_HOVER
  Constant5 : Constant  Value=0  OutDataTypeStr=single
  Constant6 : Constant  Value=MPC_THR_MAX
  Mux : Mux  Inputs=3
  Product : Product
  Saturation : Saturate  UpperLimit=1.0  LowerLimit=0.0
      settings: AttributesFormatString=[%<LowerLimit>,%<UpperLimit>]
  Saturation1 : Saturate  UpperLimit=1.0  LowerLimit=0.0
      settings: AttributesFormatString=[%<LowerLimit>,%<UpperLimit>]
  Sum : Sum  Inputs=++|
  Sum1 : Sum  Inputs=|+-
  Switch : Switch  Criteria=u2 ~= 0  SaturateOnIntegerOverflow=off  InputSameDT=off
  Switch1 : Switch  Threshold=0.5  SaturateOnIntegerOverflow=off  InputSameDT=off
  Unary Minus : UnaryMinus
  man_z_sp1 : InportShadow
  thrust_body : Outport
  wires:
  landed/1 -> Switch/2
  Constant5/1 -> Switch/1
  Switch/1 -> [throttle_min]
  Constant2/1 -> Compare To Constant/1
  Compare To Constant/1 -> Switch1/2
  Sum/1 -> Switch1/1
  [throttle_min] -> Sum/2, Sum1/2
  Constant3/1 -> Sum1/1
  Product/1 -> Sum/1
  1-D Lookup Table1/1 -> Switch1/3
  [throttle_min] -> Mux/1
  Mux/1 -> 1-D Lookup Table1/2
  Constant4/1 -> Mux/2
  Constant1/1 -> Switch/3
  man_z_sp1/1 -> Saturation/1
  Switch1/1 -> Unary Minus/1
  Unary Minus/1 -> thrust_body/1
  man_z_sp/1 -> Saturation1/1
  Sum1/1 -> Product/2
  Constant6/1 -> Mux/3
  Saturation/1 -> 1-D Lookup Table1/1
  Saturation1/1 -> Product/1

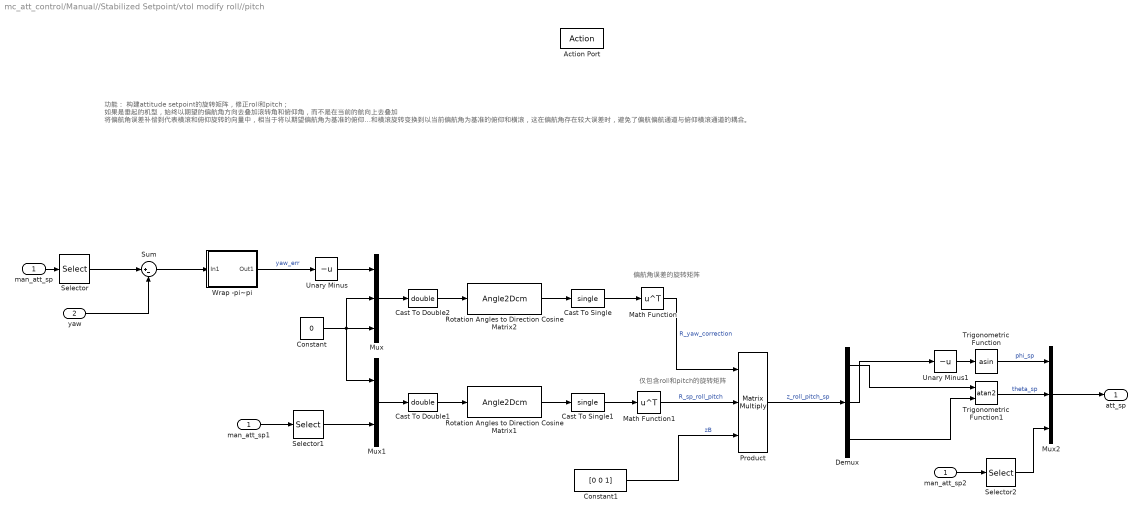
== system mc_att_control/Manual//Stabilized Setpoint/vtol modify roll//pitch ==
  note: 偏航角误差的旋转矩阵
  note: 仅包含roll和pitch的旋转矩阵
  note: 功能：
      | 构建attitude setpoint的旋转矩阵，修正roll和pitch；
      | 如果是垂起的机型，始终以期望的偏航角方向去叠加滚转角和俯仰角，而不是在当前的航向上去叠加
      | 将偏航角误差补偿到代表横滚和俯仰旋转的向量中，相当于将以期望偏航角为基准的俯仰和横滚旋转变换到以当前偏航角为基准的俯仰和横滚，这在偏航角存在较大误差时，避免了偏航偏航通道与俯仰横滚通道的耦合。
  man_att_sp : Inport
  yaw : Inport  Port=2
  Action Port : ActionPort  ActionPortLabel=if(u1 > 0)
  Cast To Double1 : DataTypeConversion  OutDataTypeStr=double  SaturateOnIntegerOverflow=off  RndMeth=Floor
  Cast To Double2 : DataTypeConversion  OutDataTypeStr=double  SaturateOnIntegerOverflow=off  RndMeth=Floor
  Cast To Single : DataTypeConversion  OutDataTypeStr=single  SaturateOnIntegerOverflow=off  RndMeth=Floor
  Cast To Single1 : DataTypeConversion  OutDataTypeStr=single  SaturateOnIntegerOverflow=off  RndMeth=Floor
  Constant : Constant  Value=0  OutDataTypeStr=single
  Constant1 : Constant  Value=[0 0 1]  OutDataTypeStr=single
  Demux : Demux  Outputs=3
  Math Function : Math  Operator=transpose
  Math Function1 : Math  Operator=transpose
  Mux : Mux  Inputs=3
  Mux1 : Mux  Inputs=2
  Mux2 : Mux  Inputs=3
  Product : Product  Inputs=3  Multiplication=Matrix(*)
  Rotation Angles to Direction Cosine Matrix1 : Angle2Dcm
      settings: AttributesFormatString=Rotation Order: %<rotationOrder>
  Rotation Angles to Direction Cosine Matrix2 : Angle2Dcm
      settings: AttributesFormatString=Rotation Order: %<rotationOrder>
  Selector : Selector  InputPortWidth=3  IndexOptions=Index vector (dialog)  Indices=3  OutputSizes=1
  Selector1 : Selector  InputPortWidth=3  IndexOptions=Index vector (dialog)  Indices=[2 1]  OutputSizes=1
  Selector2 : Selector  InputPortWidth=3  IndexOptions=Index vector (dialog)  Indices=3  OutputSizes=1
  Sum : Sum  Inputs=|+-
  Trigonometric Function : Trigonometry  Operator=asin
  Trigonometric Function1 : Trigonometry  Operator=atan2
  Unary Minus : UnaryMinus
  Unary Minus1 : UnaryMinus
  Wrap -pi~pi : Subsystem
  man_att_sp1 : InportShadow
  man_att_sp2 : InportShadow
  att_sp : Outport
  wires:
  Constant1/1 -> Product/3  "zB"
  Demux/2 -> Unary Minus1/1
  yaw/1 -> Sum/2
  Math Function1/1 -> Product/2  "R_sp_roll_pitch"
  Math Function/1 -> Product/1  "R_yaw_correction"
  Trigonometric Function1/1 -> Mux2/2  "theta_sp"
  Rotation Angles to Direction Cosine Matrix2/1 -> Cast To Single/1
  Constant/1 -> Mux1/1, Mux/2, Mux/3
  Unary Minus/1 -> Mux/1
  Mux1/1 -> Cast To Double1/1
  Mux/1 -> Cast To Double2/1
  Demux/3 -> Trigonometric Function1/2
  Demux/1 -> Trigonometric Function1/1
  Trigonometric Function/1 -> Mux2/1  "phi_sp"
  Rotation Angles to Direction Cosine Matrix1/1 -> Cast To Single1/1
  Unary Minus1/1 -> Trigonometric Function/1
  Selector/1 -> Sum/1
  Product/1 -> Demux/1  "z_roll_pitch_sp"
  Wrap -pi~pi/1(Out1) -> Unary Minus/1  "yaw_err"
  Sum/1 -> Wrap -pi~pi/1(In1)
  Cast To Double1/1 -> Rotation Angles to Direction Cosine Matrix1/1
  Cast To Double2/1 -> Rotation Angles to Direction Cosine Matrix2/1
  Selector2/1 -> Mux2/3
  Cast To Single/1 -> Math Function/1
  Cast To Single1/1 -> Math Function1/1
  man_att_sp/1 -> Selector/1
  man_att_sp1/1 -> Selector1/1
  Selector1/1 -> Mux1/2
  man_att_sp2/1 -> Selector2/1
  Mux2/1 -> att_sp/1

== system mc_att_control/Rate Control/I ==
  note: reset Integral
  note: calulate factor
  rate_err : Inport
  Compare To Constant : simulink/Logic and Bit Operations/Compare To Constant  relop=~=  const=VEHICLE_TYPE_ROTARY_WING  OutDataTypeStr=boolean
  Constant : Constant  Value=[0 0 0]  OutDataTypeStr=single
  Discrete-Time Integrator : DiscreteIntegrator  ExternalReset=level  SampleTime=-1  LimitOutput=on  UpperSaturationLimit=[MC_RR_INT_LIM, MC_PR_INT_LIM, MC_YR_INT_LIM]  LowerSaturationLimit=-[MC_RR_INT_LIM, MC_PR_INT_LIM, MC_YR_INT_LIM]  ICPrevOutput=DiscIntNeverNeededParam  ICPrevScaledInput=DiscIntNeverNeededParam
      settings: AttributesFormatString=|
      | %<LowerSaturationLimit>
      | %<UpperSaturationLimit>
  Gain : Gain  Gain=[MC_ROLLRATE_K*MC_ROLLRATE_I, MC_PITCHRATE_K*MC_PITCHRATE_I, MC_YAWRATE_K*MC_YAWRATE_I]
      settings: AttributesFormatString=%<Gain>
  Gain2 : Gain  Gain=1/deg2rad(400)
      settings: AttributesFormatString=%<Gain>
  I2 : Constant  Value=[1 1 1]  OutDataTypeStr=single
  I3 : Constant  Value=[0 0 0]  OutDataTypeStr=single
  Logical Operator : Logic  Operator=OR  AllPortsSameDT=off  OutDataTypeStr=boolean
  Logical Operator2 : Logic  Operator=NOT  AllPortsSameDT=off  OutDataTypeStr=boolean
  Max : MinMax  Function=max  Inputs=2
  Product : Product
  Square : Math  Operator=square
  Sum : Sum  Inputs=|+-
  Switch : Switch  Criteria=u2 ~= 0  SaturateOnIntegerOverflow=off  InputSameDT=off
  mixer saturation : Subsystem
  rate_I : Outport
  wires:
  [rate_err] -> Gain2/1
  I2/1 -> Sum/1
  Square/1 -> Sum/2
  Sum/1 -> Max/2
  I3/1 -> Max/1
  Product/1 -> Switch/3
  Gain/1 -> Product/1
  Max/1 -> Product/2
  Discrete-Time Integrator/1 -> rate_I/1
  mixer saturation/1(rate_err_limited) -> [rate_err], Gain/1
  rate_err/1 -> mixer saturation/1(rate_err)
  [whether_landed] -> Switch/2
  Constant/1 -> Switch/1
  Switch/1 -> Discrete-Time Integrator/1
  [vehicle_type] -> Compare To Constant/1
  Compare To Constant/1 -> Logical Operator/2
  [flag_armed] -> Logical Operator2/1
  Logical Operator2/1 -> Logical Operator/1
  Logical Operator/1 -> Discrete-Time Integrator/2
  Gain2/1 -> Square/1  "i_factor"

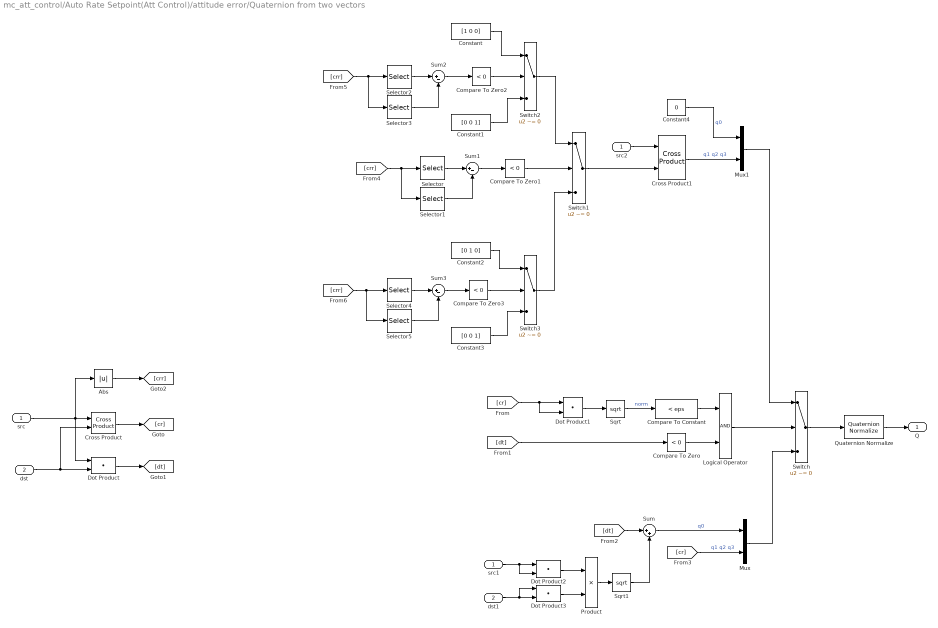
== system mc_att_control/Auto Rate Setpoint(Att Control)/attitude error/Quaternion from two vectors ==
  src : Inport
  dst : Inport  Port=2
  Abs : Abs  SaturateOnIntegerOverflow=off
  Compare To Constant : simulink/Logic and Bit Operations/Compare To Constant  relop=<  const=eps  OutDataTypeStr=boolean
  Compare To Zero{,1..3} (4 alike) : simulink/Logic and Bit Operations/Compare To Zero  relop=<  OutDataTypeStr=boolean
  Constant : Constant  Value=[1 0 0]  OutDataTypeStr=single
  Constant1 : Constant  Value=[0 0 1]  OutDataTypeStr=single
  Constant2 : Constant  Value=[0 1 0]  OutDataTypeStr=single
  Constant3 : Constant  Value=[0 0 1]  OutDataTypeStr=single
  Constant4 : Constant  Value=0  OutDataTypeStr=single
  Cross Product : vrlib/Utilities/Cross Product
  Cross Product1 : vrlib/Utilities/Cross Product
  Dot Product{,1..3} (4 alike) : DotProduct  OutDataTypeStr=Inherit: Inherit via internal rule
  Logical Operator : Logic  AllPortsSameDT=off  OutDataTypeStr=boolean
  Mux : Mux  Inputs=2
  Mux1 : Mux  Inputs=2
  Product : Product
  Quaternion Normalize : sharedutil/Quaternion Normalize  aMode=aMode
  Selector : Selector  InputPortWidth=3  IndexOptions=Index vector (dialog)  Indices=1  OutputSizes=1
  Selector1 : Selector  InputPortWidth=3  IndexOptions=Index vector (dialog)  Indices=2  OutputSizes=1
  Selector2 : Selector  InputPortWidth=3  IndexOptions=Index vector (dialog)  Indices=1  OutputSizes=1
  Selector3 : Selector  InputPortWidth=3  IndexOptions=Index vector (dialog)  Indices=3  OutputSizes=1
  Selector4 : Selector  InputPortWidth=3  IndexOptions=Index vector (dialog)  Indices=2  OutputSizes=1
  Selector5 : Selector  InputPortWidth=3  IndexOptions=Index vector (dialog)  Indices=3  OutputSizes=1
  Sqrt : Sqrt
  Sqrt1 : Sqrt
  Sum : Sum  Inputs=|++
  Sum1 : Sum  Inputs=|+-
  Sum2 : Sum  Inputs=|+-
  Sum3 : Sum  Inputs=|+-
  Switch{,1..3} (4 alike) : Switch  Criteria=u2 ~= 0  SaturateOnIntegerOverflow=off  InputSameDT=off
  dst1 : InportShadow  Port=2
  src1 : InportShadow
  src2 : InportShadow
  Q : Outport
  wires:
  src/1 -> Abs/1, Dot Product/1, Cross Product/1
  dst/1 -> Dot Product/2, Cross Product/2
  [cr] -> Dot Product1/2, Dot Product1/1
  [dt] -> Compare To Zero/1
  Dot Product1/1 -> Sqrt/1
  Sqrt/1 -> Compare To Constant/1  "norm"
  Compare To Constant/1 -> Logical Operator/1
  Compare To Zero/1 -> Logical Operator/2
  Logical Operator/1 -> Switch/2
  Cross Product/1 -> [cr]
  Dot Product/1 -> [dt]
  [dt] -> Sum/1
  Sqrt1/1 -> Sum/2
  Sum/1 -> Mux/1  "q0"
  Product/1 -> Sqrt1/1
  Dot Product2/1 -> Product/1
  src1/1 -> Dot Product2/2, Dot Product2/1
  Dot Product3/1 -> Product/2
  dst1/1 -> Dot Product3/1, Dot Product3/2
  [cr] -> Mux/2  "q1 q2 q3"
  Mux/1 -> Switch/3
  Switch/1 -> Quaternion Normalize/1
  Quaternion Normalize/1 -> Q/1
  Abs/1 -> [crr]
  Selector/1 -> Sum1/1
  [crr] -> Selector/1, Selector1/1
  Selector1/1 -> Sum1/2
  Sum1/1 -> Compare To Zero1/1
  Compare To Zero1/1 -> Switch1/2
  Switch2/1 -> Switch1/1
  Sum2/1 -> Compare To Zero2/1
  Selector3/1 -> Sum2/2
  [crr] -> Selector3/1, Selector2/1
  Selector2/1 -> Sum2/1
  Compare To Zero2/1 -> Switch2/2
  Constant/1 -> Switch2/1
  Constant1/1 -> Switch2/3
  Selector4/1 -> Sum3/1
  [crr] -> Selector4/1, Selector5/1
  Selector5/1 -> Sum3/2
  Sum3/1 -> Compare To Zero3/1
  Compare To Zero3/1 -> Switch3/2
  Constant2/1 -> Switch3/1
  Constant3/1 -> Switch3/3
  Switch3/1 -> Switch1/3
  Switch1/1 -> Cross Product1/2
  src2/1 -> Cross Product1/1
  Cross Product1/1 -> Mux1/2  "q1 q2 q3"
  Constant4/1 -> Mux1/1  "q0"
  Mux1/1 -> Switch/1

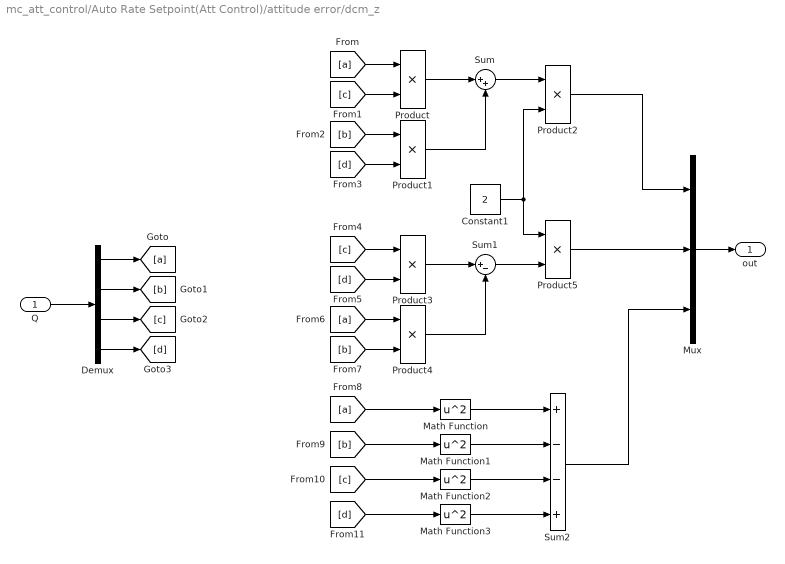
== system mc_att_control/Auto Rate Setpoint(Att Control)/attitude error/dcm_z ==
  Q : Inport
  Constant1 : Constant  Value=2  OutDataTypeStr=single
  Demux : Demux
  Math Function{,1..3} (4 alike) : Math  Operator=square
  Mux : Mux  Inputs=3
  Product{,1..5} (6 alike) : Product
  Sum : Sum  Inputs=|++
  Sum1 : Sum  Inputs=|+-
  Sum2 : Sum  Inputs=+--+
  out : Outport
  wires:
  Q/1 -> Demux/1
  Demux/1 -> [a]
  Demux/2 -> [b]
  Demux/3 -> [c]
  Demux/4 -> [d]
  [a] -> Product/1
  [c] -> Product/2
  Product/1 -> Sum/1
  [b] -> Product1/1
  [d] -> Product1/2
  Product1/1 -> Sum/2
  Sum/1 -> Product2/1
  Product2/1 -> Mux/1
  Mux/1 -> out/1
  [c] -> Product3/1
  [d] -> Product3/2
  Product3/1 -> Sum1/1
  [a] -> Product4/1
  [b] -> Product4/2
  Product4/1 -> Sum1/2
  Sum1/1 -> Product5/2
  Constant1/1 -> Product5/1, Product2/2
  Product5/1 -> Mux/2
  Sum2/1 -> Mux/3
  [a] -> Math Function/1
  [b] -> Math Function1/1
  [c] -> Math Function2/1
  [d] -> Math Function3/1
  Math Function/1 -> Sum2/1
  Math Function1/1 -> Sum2/2
  Math Function2/1 -> Sum2/3
  Math Function3/1 -> Sum2/4

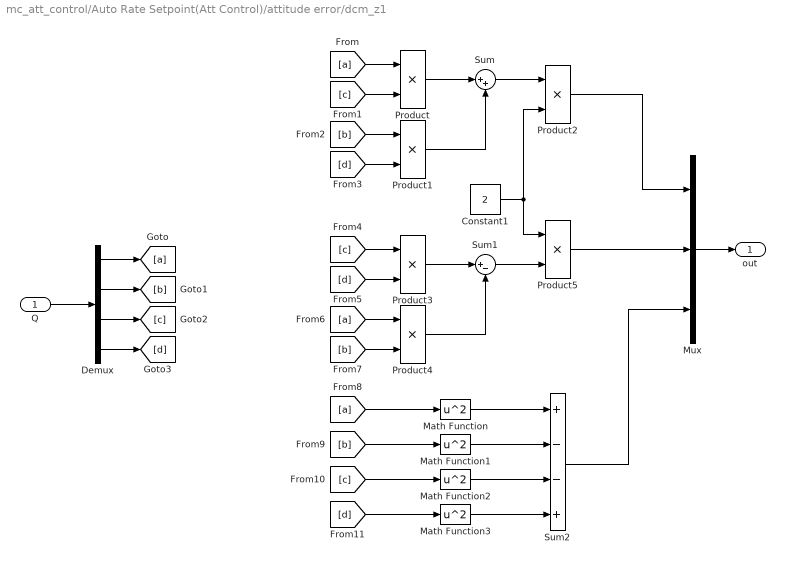
== system mc_att_control/Auto Rate Setpoint(Att Control)/attitude error/dcm_z1 ==
  Q : Inport
  Constant1 : Constant  Value=2  OutDataTypeStr=single
  Demux : Demux
  Math Function{,1..3} (4 alike) : Math  Operator=square
  Mux : Mux  Inputs=3
  Product{,1..5} (6 alike) : Product
  Sum : Sum  Inputs=|++
  Sum1 : Sum  Inputs=|+-
  Sum2 : Sum  Inputs=+--+
  out : Outport
  wires:
  Math Function3/1 -> Sum2/4
  Math Function2/1 -> Sum2/3
  Math Function1/1 -> Sum2/2
  Math Function/1 -> Sum2/1
  [d] -> Math Function3/1
  [c] -> Math Function2/1
  [b] -> Math Function1/1
  [a] -> Math Function/1
  Sum2/1 -> Mux/3
  Product5/1 -> Mux/2
  Constant1/1 -> Product2/2, Product5/1
  Sum1/1 -> Product5/2
  Product4/1 -> Sum1/2
  [b] -> Product4/2
  [a] -> Product4/1
  Product3/1 -> Sum1/1
  [d] -> Product3/2
  [c] -> Product3/1
  Mux/1 -> out/1
  Product2/1 -> Mux/1
  Sum/1 -> Product2/1
  Product1/1 -> Sum/2
  [d] -> Product1/2
  [b] -> Product1/1
  Product/1 -> Sum/1
  [c] -> Product/2
  [a] -> Product/1
  Demux/4 -> [d]
  Demux/3 -> [c]
  Demux/2 -> [b]
  Demux/1 -> [a]
  Q/1 -> Demux/1

== system mc_att_control/Manual//Stabilized Setpoint/man_yaw_sp/Wrap -pi~pi ==
  In1 : Inport
  Bias : Bias  Bias=pi  SaturateOnIntegerOverflow=off
  Bias1 : Bias  Bias=-pi  SaturateOnIntegerOverflow=off
  Constant1 : Constant  Value=2*pi  OutDataTypeStr=single
  Mod : Math  Operator=mod
  man_yaw_sp : Outport
  wires:
  Constant1/1 -> Mod/2
  Mod/1 -> Bias1/1
  In1/1 -> Bias/1
  Bias/1 -> Mod/1
  Bias1/1 -> man_yaw_sp/1

== system mc_att_control/Manual//Stabilized Setpoint/mapping for roll& pitch setpoint/AxisAngle to Quat ==
  note: 轴角法转四元数
      | $vect = [u, v, w] = |vect| \cdot n \\ angle为[u, v, w] \text{合成的角度} \\ quat = [\cos(\frac{| angle |}{2}), \sin(\frac{| angle |}{2}) \cdot n]$
  AxisAngle1 : Inport
  Constant1 : Constant  Value=0  OutDataTypeStr=single
  Constant2 : Constant  Value=[1 0 0 0]  OutDataTypeStr=single
  Cos : Trigonometry  Operator=cos
  Divide1 : Product  Inputs=*/
  Dot Product : DotProduct  OutDataTypeStr=Inherit: Inherit via internal rule
  Gain1 : Gain  Gain=0.5
  Mux2 : Mux  Inputs=2
  Mux3 : Mux  Inputs=2
  Product1 : Product
  Sin : Trigonometry
  Sqrt1 : Sqrt
  Switch : Switch  Criteria=u2 > Threshold  Threshold=eps  SaturateOnIntegerOverflow=off  InputSameDT=off
  Quat : Outport
  wires:
  Constant1/1 -> Mux3/2
  Gain1/1 -> Sin/1, Cos/1
  Mux3/1 -> Dot Product/2, Dot Product/1, Divide1/1  "q_sp_rpy"
  Cos/1 -> Mux2/1  "q0"
  AxisAngle1/1 -> Mux3/1
  Product1/1 -> Mux2/2
  Sin/1 -> Product1/1  "magnitude"
  Divide1/1 -> Product1/2  "axis"
  Switch/1 -> Quat/1
  Mux2/1 -> Switch/1
  Sqrt1/1 -> Switch/2, Divide1/2, Gain1/1  "angle"
  Dot Product/1 -> Sqrt1/1
  Constant2/1 -> Switch/3
